simulink subsystem "Eulerr"  (R2020a)
settings: Solver=VariableStepAuto  StartTime=0.0  StopTime=10.0  RelTol=1e-3
settings Model: Creator=verti  LastModifiedBy=verti
settings DebuggingCC: SFMachineParentedDataDiag=error

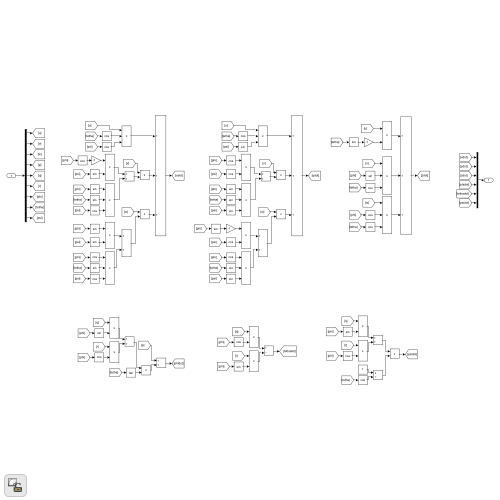
[thumbnail: Simulink's stored preview of the top-level diagram]
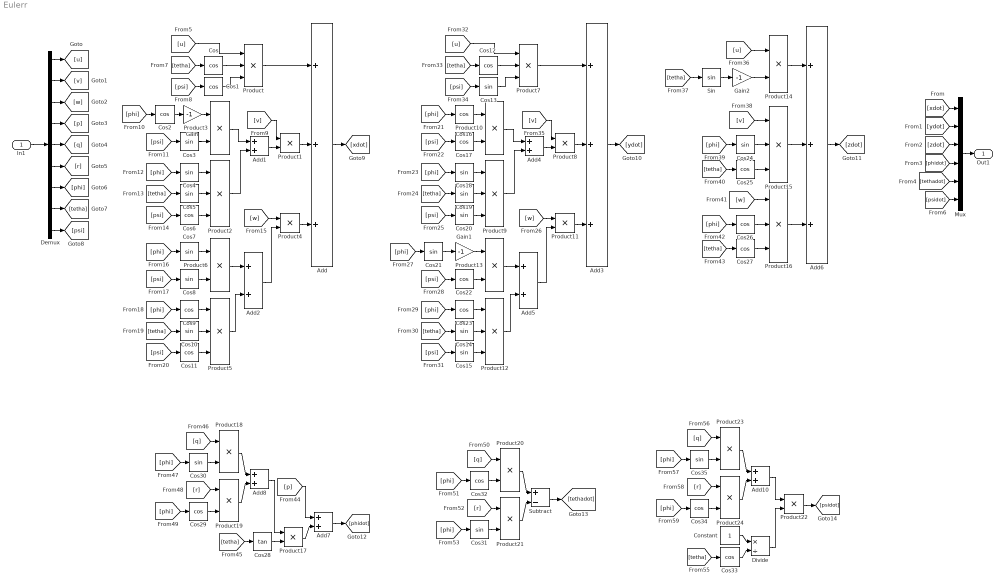
== system Eulerr ==
  In1 : Inport  RequirementInfo={} %GIDa_30f44a4e_08d4_4601_93c3_dd5dc3ba1d66
  Add : Sum  RequirementInfo={} %GIDa_aefd7acc_b93c_43ef_bc22_93173b15d26a  Inputs=+++
  Add1 : Sum  RequirementInfo={} %GIDa_1df7e404_709f_4c34_bfb1_9edb86e0933e
  Add10 : Sum  RequirementInfo={} %GIDa_5736c293_6e8c_4e62_93e1_8587205b4de4
  Add2 : Sum  RequirementInfo={} %GIDa_7408d37c_c07e_40d2_a8d3_f67b083cd7a6
  Add3 : Sum  RequirementInfo={} %GIDa_9bc6c77d_00b8_4be2_9998_9f383e2ec964  Inputs=+++
  Add4 : Sum  RequirementInfo={} %GIDa_27ee5c98_b771_4e62_92da_e735bb30a9f1
  Add5 : Sum  RequirementInfo={} %GIDa_0dfd2260_03ad_4d91_86ac_cd9b324daccd
  Add6 : Sum  RequirementInfo={} %GIDa_3c8e3aa9_1a02_4a99_aec8_7a1d4531d47e  Inputs=+++
  Add7 : Sum  RequirementInfo={} %GIDa_3e86a3f6_2cb5_4d50_a628_c17e44f19cfc
  Add8 : Sum  RequirementInfo={} %GIDa_35ded7ae_5e19_4872_9ee4_1b18323c952f
  Constant : Constant  RequirementInfo={} %GIDa_023206b9_6b61_431f_9830_5c891cdd6bd7
  Cos : Trigonometry  RequirementInfo={} %GIDa_cac46dec_d3d5_45d7_ae5a_8e2245639bdf  Operator=cos
  Cos1 : Trigonometry  RequirementInfo={} %GIDa_a2affaf6_7c96_4525_bac9_12a998858108  Operator=cos
  Cos10 : Trigonometry  RequirementInfo={} %GIDa_18c678f3_f379_4ab8_b91b_562aa38c16e2
  Cos11 : Trigonometry  RequirementInfo={} %GIDa_0efc8b24_5e40_4ccb_998a_e1d942741ad9  Operator=cos
  Cos12 : Trigonometry  RequirementInfo={} %GIDa_9d12c00d_9d5d_4ba4_baec_2d4bfac5175b  Operator=cos
  Cos13 : Trigonometry  RequirementInfo={} %GIDa_c6021834_267a_437a_8b30_a77688bd744a
  Cos14 : Trigonometry  RequirementInfo={} %GIDa_db539042_8ae7_4920_9cad_cd07c116c5c2
  Cos15 : Trigonometry  RequirementInfo={} %GIDa_4050018a_e8a1_40c4_8a25_e724c39ac556
  Cos16 : Trigonometry  RequirementInfo={} %GIDa_897af14b_b122_4e7e_9c59_2b472178e807  Operator=cos
  Cos17 : Trigonometry  RequirementInfo={} %GIDa_6549ba05_29df_49cd_89a7_99aa525f7b47  Operator=cos
  Cos18 : Trigonometry  RequirementInfo={} %GIDa_9a70300a_6eb1_45d1_92a9_b202009084c5
  Cos19 : Trigonometry  RequirementInfo={} %GIDa_62d2849f_7d58_4e19_a9c0_175b63678cb2
  Cos2 : Trigonometry  RequirementInfo={} %GIDa_36ad0073_a0e6_4e40_afac_4072bb478f07  Operator=cos
  Cos20 : Trigonometry  RequirementInfo={} %GIDa_f61faac6_6442_4523_9c21_b1d2f5c6d4b3
  Cos21 : Trigonometry  RequirementInfo={} %GIDa_184a00ce_f7db_4840_a738_c707251738e2
  Cos22 : Trigonometry  RequirementInfo={} %GIDa_cf971a71_24c7_4c17_a117_337ab9424feb  Operator=cos
  Cos23 : Trigonometry  RequirementInfo={} %GIDa_e2c4cb53_8ecf_4864_9b71_61a426d1e062  Operator=cos
  Cos24 : Trigonometry  RequirementInfo={} %GIDa_5f7b61b2_270f_4d19_9352_711e2da6f8b0
  Cos25 : Trigonometry  RequirementInfo={} %GIDa_f535e83d_0792_45a2_9d9a_abb8603ede90  Operator=cos
  Cos26 : Trigonometry  RequirementInfo={} %GIDa_088b62a8_203e_4a9c_b639_f580891f8099  Operator=cos
  Cos27 : Trigonometry  RequirementInfo={} %GIDa_a0a543e9_ddfa_4b54_ab61_a3c71a3070da  Operator=cos
  Cos28 : Trigonometry  RequirementInfo={} %GIDa_68181c4f_a5ed_4d3e_b33c_cbe77b92d732  Operator=tan
  Cos29 : Trigonometry  RequirementInfo={} %GIDa_2210e1b3_de7f_4802_b8e9_18a0113c1c90  Operator=cos
  Cos3 : Trigonometry  RequirementInfo={} %GIDa_1b551447_5960_4e96_82d3_6b09fb8f7e4c
  Cos30 : Trigonometry  RequirementInfo={} %GIDa_062ac2f7_7d4e_4650_ae63_9eef4048f879
  Cos31 : Trigonometry  RequirementInfo={} %GIDa_5dd55b76_8c78_45ad_a7fa_b22aae851f7a
  Cos32 : Trigonometry  RequirementInfo={} %GIDa_905621b8_220b_44ac_9430_5ffc0213d97f  Operator=cos
  Cos33 : Trigonometry  RequirementInfo={} %GIDa_92c930dc_9b71_4c46_afef_fab97cdabd7d  Operator=cos
  Cos34 : Trigonometry  RequirementInfo={} %GIDa_8495fd9a_cde0_4200_b34f_0ff00a2209d1  Operator=cos
  Cos35 : Trigonometry  RequirementInfo={} %GIDa_617eb6c0_6936_48e9_97e1_ea165c6ef812
  Cos4 : Trigonometry  RequirementInfo={} %GIDa_7778c288_8828_42b2_9e74_dcae5b59cf99
  Cos5 : Trigonometry  RequirementInfo={} %GIDa_a83a07c9_8e51_43d5_97a8_34dd1a336b25
  Cos6 : Trigonometry  RequirementInfo={} %GIDa_11cd9b5f_221b_4b01_84fc_5d39c765ce90  Operator=cos
  Cos7 : Trigonometry  RequirementInfo={} %GIDa_8c5b1670_ce36_46e1_a144_c4f54314b35b
  Cos8 : Trigonometry  RequirementInfo={} %GIDa_0e3abf51_dd7a_40a0_be78_a20732ae564c
  Cos9 : Trigonometry  RequirementInfo={} %GIDa_6d104f46_4ee9_4e03_8061_4c1a09ca8730  Operator=cos
  Demux : Demux  RequirementInfo={} %GIDa_75e6b640_0ed9_4149_a79b_6af24c540d0c  Outputs=9
  Divide : Product  RequirementInfo={} %GIDa_60eb3dfd_bd8c_4e24_979c_6797a11c3044  Inputs=*/
  Gain : Gain  RequirementInfo={} %GIDa_54efdb4a_84af_47b5_8948_42588eb79462  Gain=-1
  Gain1 : Gain  RequirementInfo={} %GIDa_0981faac_2b38_4d21_a0d5_e3ca153480c5  Gain=-1
  Gain2 : Gain  RequirementInfo={} %GIDa_033048aa_224e_46d6_b317_c240a9245122  Gain=-1
  Mux : Mux  RequirementInfo={} %GIDa_fd738df3_59e5_4359_87b7_55dce8a3149d  Inputs=6
  Product : Product  RequirementInfo={} %GIDa_eac7b197_7a63_4a5d_b11f_1c09220a0f9f  Inputs=3
  Product1 : Product  RequirementInfo={} %GIDa_b51841df_a252_45e4_888a_d06fe367d5e2
  Product10 : Product  RequirementInfo={} %GIDa_2329422e_ea94_43f3_8fda_a7d68348db79
  Product11 : Product  RequirementInfo={} %GIDa_acb239ac_fc6c_43e0_9475_eeecc4e8de3d
  Product12 : Product  RequirementInfo={} %GIDa_e656d79c_c4e2_44f9_acba_c5a6e6749feb  Inputs=3
  Product13 : Product  RequirementInfo={} %GIDa_571bee9e_c83c_4a23_ae72_72baa9beaea6
  Product14 : Product  RequirementInfo={} %GIDa_12684f0f_f9cc_49dd_ba5c_c3dd201aeebd
  Product15 : Product  RequirementInfo={} %GIDa_736c4fdf_95d0_4694_a633_67ed18dea77e  Inputs=3
  Product16 : Product  RequirementInfo={} %GIDa_2840d212_5245_4366_875d_9b1a33c35ed1  Inputs=3
  Product17 : Product  RequirementInfo={} %GIDa_08920c1e_9838_48b9_a39b_255e35cc11bc
  Product18 : Product  RequirementInfo={} %GIDa_0bab1363_8081_48f9_81e9_d06d9516b49c
  Product19 : Product  RequirementInfo={} %GIDa_a34f626b_12ea_4595_9a12_7e1f593343a0
  Product2 : Product  RequirementInfo={} %GIDa_73f4bf5d_b5e6_4064_8f0d_bdc4601980fe  Inputs=3
  Product20 : Product  RequirementInfo={} %GIDa_bebd23e9_4d42_4c60_bd75_826d302497bf
  Product21 : Product  RequirementInfo={} %GIDa_3bbe0df2_ec56_47e6_b2a6_5d5cbc210fa8
  Product22 : Product  RequirementInfo={} %GIDa_4ab4540d_6779_40d2_99e1_dad7077285eb
  Product23 : Product  RequirementInfo={} %GIDa_b5e55469_f7fb_450d_b600_1a8cb62f30b8
  Product24 : Product  RequirementInfo={} %GIDa_20ee402b_8f20_4ac7_9853_7cff53a912f3
  Product3 : Product  RequirementInfo={} %GIDa_33294ef1_2301_4f82_ad6e_65d766a1bcb7
  Product4 : Product  RequirementInfo={} %GIDa_4e36938b_643e_44ab_96ab_b4d9d5e242c3
  Product5 : Product  RequirementInfo={} %GIDa_46665cd3_8854_495a_ae17_6823c2268420  Inputs=3
  Product6 : Product  RequirementInfo={} %GIDa_92445a7b_0e87_4834_b5c2_5e8615aa1ddd
  Product7 : Product  RequirementInfo={} %GIDa_0c3f5330_c9e0_4851_9386_35fb2c46e43a  Inputs=3
  Product8 : Product  RequirementInfo={} %GIDa_9404c120_6282_44e5_8470_e343d01f8f0f
  Product9 : Product  RequirementInfo={} %GIDa_302b394d_ddcc_4fee_a995_5e35f0d60e1f  Inputs=3
  Sin : Trigonometry  RequirementInfo={} %GIDa_69fe2085_3876_489f_af13_b9d3a41c5399
  Subtract : Sum  RequirementInfo={} %GIDa_050071f0_4b3b_4350_b8fd_9acf5bf5a5fc  Inputs=+-
  Out1 : Outport  RequirementInfo={} %GIDa_b62859c1_eeb4_4a43_b617_dc3f70d6ea8a
  wires:
  In1/1 -> Demux/1
  Demux/1 -> [u]
  Demux/2 -> [v]
  Demux/3 -> [w]
  Demux/4 -> [p]
  Demux/5 -> [q]
  Demux/6 -> [r]
  Demux/7 -> [phi]
  Demux/8 -> [tetha]
  Demux/9 -> [psi]
  Mux/1 -> Out1/1
  [xdot] -> Mux/1
  [ydot] -> Mux/2
  [tethadot] -> Mux/5
  [psidot] -> Mux/6
  [phidot] -> Mux/4
  [zdot] -> Mux/3
  Add/1 -> [xdot]
  [psi] -> Cos1/1
  [tetha] -> Cos/1
  Cos1/1 -> Product/3
  Cos/1 -> Product/2
  [u] -> Product/1
  Product/1 -> Add/1
  Product1/1 -> Add/2
  [v] -> Product1/1
  Add1/1 -> Product1/2
  Product2/1 -> Add1/2
  Product3/1 -> Add1/1
  [phi] -> Cos2/1
  Cos2/1 -> Gain/1
  Gain/1 -> Product3/1
  Cos3/1 -> Product3/2
  [psi] -> Cos3/1
  [phi] -> Cos4/1
  [tetha] -> Cos5/1
  [psi] -> Cos6/1
  Cos5/1 -> Product2/2
  Cos4/1 -> Product2/1
  Cos6/1 -> Product2/3
  Add2/1 -> Product4/2
  [w] -> Product4/1
  Product4/1 -> Add/3
  Cos11/1 -> Product5/3
  Cos9/1 -> Product5/1
  Cos10/1 -> Product5/2
  [psi] -> Cos11/1
  [tetha] -> Cos10/1
  [phi] -> Cos9/1
  [psi] -> Cos8/1
  Cos8/1 -> Product6/2
  Cos7/1 -> Product6/1
  [phi] -> Cos7/1
  Product6/1 -> Add2/1
  Product5/1 -> Add2/2
  Product12/1 -> Add5/2
  Product13/1 -> Add5/1
  [phi] -> Cos21/1
  Cos21/1 -> Gain1/1
  Cos22/1 -> Product13/2
  [psi] -> Cos22/1
  [phi] -> Cos23/1
  [tetha] -> Cos14/1
  [psi] -> Cos15/1
  Cos14/1 -> Product12/2
  Cos23/1 -> Product12/1
  Cos15/1 -> Product12/3
  Product11/1 -> Add3/3
  [w] -> Product11/1
  Add5/1 -> Product11/2
  Cos20/1 -> Product9/3
  Cos18/1 -> Product9/1
  Cos19/1 -> Product9/2
  [psi] -> Cos20/1
  [tetha] -> Cos19/1
  [phi] -> Cos18/1
  [psi] -> Cos17/1
  Cos17/1 -> Product10/2
  Cos16/1 -> Product10/1
  [phi] -> Cos16/1
  Product10/1 -> Add4/1
  Product9/1 -> Add4/2
  Add4/1 -> Product8/2
  [v] -> Product8/1
  Product8/1 -> Add3/2
  Product7/1 -> Add3/1
  [u] -> Product7/1
  Cos12/1 -> Product7/2
  Cos13/1 -> Product7/3
  [tetha] -> Cos12/1
  [psi] -> Cos13/1
  Add3/1 -> [ydot]
  Gain1/1 -> Product13/1
  Add6/1 -> [zdot]
  Product14/1 -> Add6/1
  [u] -> Product14/1
  [tetha] -> Sin/1
  Sin/1 -> Gain2/1
  Gain2/1 -> Product14/2
  Product15/1 -> Add6/2
  [v] -> Product15/1
  [phi] -> Cos24/1
  [tetha] -> Cos25/1
  Cos25/1 -> Product15/3
  Cos24/1 -> Product15/2
  Cos26/1 -> Product16/2
  Cos27/1 -> Product16/3
  [tetha] -> Cos27/1
  [phi] -> Cos26/1
  [w] -> Product16/1
  Product16/1 -> Add6/3
  Add7/1 -> [phidot]
  [p] -> Add7/1
  Product17/1 -> Add7/2
  Add8/1 -> Product17/1
  [tetha] -> Cos28/1
  Cos28/1 -> Product17/2
  [q] -> Product18/1
  Cos30/1 -> Product18/2
  [phi] -> Cos30/1
  Product18/1 -> Add8/1
  [phi] -> Cos29/1
  Cos29/1 -> Product19/2
  [r] -> Product19/1
  Product19/1 -> Add8/2
  Product21/1 -> Subtract/2
  [r] -> Product21/1
  Cos31/1 -> Product21/2
  [phi] -> Cos31/1
  Product20/1 -> Subtract/1
  [phi] -> Cos32/1
  Cos32/1 -> Product20/2
  [q] -> Product20/1
  Subtract/1 -> [tethadot]
  Product24/1 -> Add10/2
  [r] -> Product24/1
  Cos34/1 -> Product24/2
  [phi] -> Cos34/1
  Product23/1 -> Add10/1
  [phi] -> Cos35/1
  Cos35/1 -> Product23/2
  [q] -> Product23/1
  [tetha] -> Cos33/1
  Add10/1 -> Product22/1
  Product22/1 -> [psidot]
  Constant/1 -> Divide/1
  Cos33/1 -> Divide/2
  Divide/1 -> Product22/2
